simulink model "model — kopia — kopia"  (R2020b)
settings: Solver=VariableStepAuto  StartTime=0.0  StopTime=20000  MaxStep=5  RelTol=1e-3
values from neighbouring files (symbols this model uses):
  A = zeros(2)    [m1 — kopia.m]    (also in model.m)
  B = zeros(2)    [m1 — kopia.m]    (also in model.m)
  Cvg = Cpo*ROo*0.005    (= 14400)    [m1 — kopia.m]    (also in model.m = 14.4)
  Cvw = Cpp*ROp*60    (= 72360)    [m1 — kopia.m]    (also in model.m = 120600)
  dqg = 0 * qg0    (= 0)    [m1 — kopia.m]    (also in model.m = 200)
  dTwew = 0    [m1 — kopia.m]
  dTzew = 3    [m1 — kopia.m]    (also in model.m = 0)
  init_con = [Twew0;Tg0]    [m1 — kopia.m]    (also in model.m = [Twew;Tg])
  k = 5    [m1 — kopia.m]
  Kcg = qg0/(Tg0-Twew0)    (= 100)    [m1 — kopia.m]    (also in model.m)
  Kcw = qg0/(Twew0-Tzew0)    (= 50)    [m1 — kopia.m]    (also in model.m)
  Kp = 0.9*T/(k*T0)    (= 0.46008109478)    [m1 — kopia.m]
  L1 = Kcg    (= 100)    [m1 — kopia.m]    (also in model.m)
  L2 = [Cvg*Kcw,Kcg*Kcw]    [m1 — kopia.m]    (also in model.m)
  L3 = [Cvw,Kcg+Kcw]    [m1 — kopia.m]    (also in model.m)
  L4 = Kcg*Kcw    (= 5000)    [m1 — kopia.m]    (also in model.m)
  M1 = [Cvw*Cvg,Cvg*(Kcg+Kcw)+Cvw*Kcg,Kcw*Kcg]    [m1 — kopia.m]    (also in model.m)
  qg0 = qgN * 1.0    (= 2000)    [m1 — kopia.m]    (also in model.m)
  stepTime = 1000    [m1 — kopia.m]    (also in model.m)
  T = 2521.5    [m1 — kopia.m]
  T0 = 986.5    [m1 — kopia.m]
  Tg = 40    [model.m]
  Ti = 3.33*T0    (= 3285.045)    [m1 — kopia.m]
  Twew = 20    [model.m]
  Twew0 = 20    [m1 — kopia.m]
  Twew_zadana = Twew0    (= 20)    [m1 — kopia.m]
  Tzew0 = TzewN + 0    (= -20)    [m1 — kopia.m]    (also in model.m)
settings Model: OrderedModelArguments=off  Creator=Lab320  LastModifiedBy=Lab320

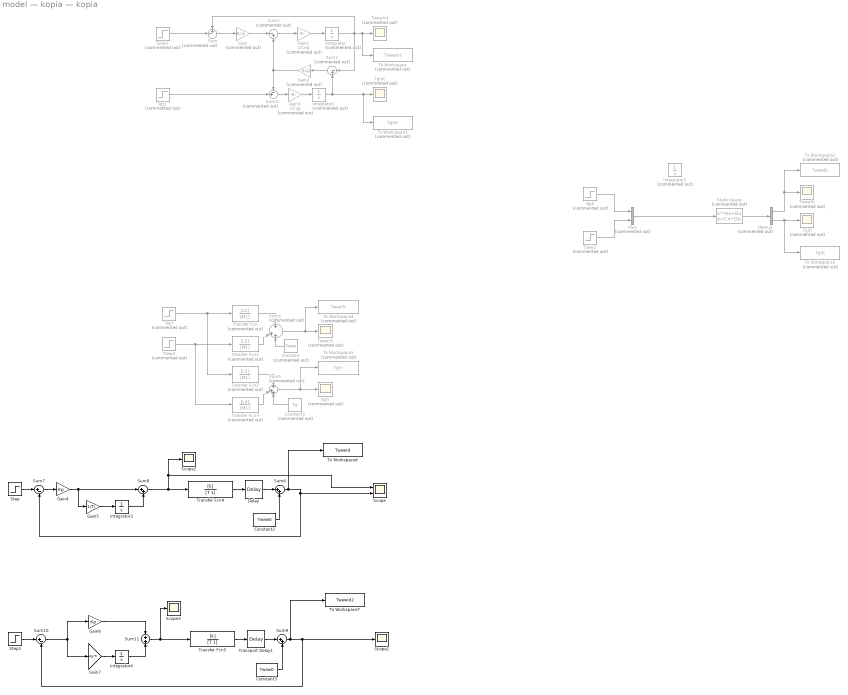
== system model — kopia — kopia ==
  " Delay" : TransportDelay  DelayTime=T0
  Constant : Constant  Commented=on  Value=Twew
  Constant1 : Constant  Commented=on  Value=Tg
  Constant2 : Constant  Value=Twew0
  Constant3 : Constant  Value=Twew0
  Demux : Demux  Commented=on  Outputs=2
  Gain : Gain  Commented=on  Gain=Kcw
  Gain1 : Gain  Commented=on  Gain=1/Cvw
  Gain2 : Gain  Commented=on  Gain=Kcg
  Gain3 : Gain  Commented=on  Gain=1/Cvg
  Gain4 : Gain  Gain=Kp
  Gain5 : Gain  Gain=1/Ti
  Gain6 : Gain  Gain=Kp
  Gain7 : Gain  Gain=Kp/Ti
  Integrator : Integrator  Commented=on  InitialCondition=Twew
  Integrator1 : Integrator  Commented=on  InitialCondition=Tg
  Integrator2 : Integrator  Commented=on
  Integrator3 : Integrator
  Integrator4 : Integrator
  Mux : Mux  Commented=on  Inputs=2
  Qg1 : Step  Commented=on  Time=stepTime  Before=qg0  After=qg0+dqg  SampleTime=0
  Qg2 : Step  Commented=on  Time=stepTime  Before=qg0  After=qg0+dqg  SampleTime=0
  Qg3 : Step  Commented=on  Time=stepTime  After=dqg  SampleTime=0
  Scope : Scope  NumInputPorts=2
  Scope1 : Scope
  Scope2 : Scope
  Scope3 : Scope
  State-Space : StateSpace  Commented=on  A=A  B=B  C=[1,0;0,1]  D=[0,0;0,0]  InitialCondition=init_con
  Step : Step  Time=0  Before=Twew_zadana  After=Twew_zadana+dTwew  SampleTime=0
  Step1 : Step  Time=stepTime  Before=Twew_zadana  After=Twew_zadana+dTwew  SampleTime=0
  Sum : Sum  Commented=on  Inputs=+-|
  Sum1 : Sum  Commented=on  Inputs=|-+
  Sum10 : Sum  Inputs=|+-
  Sum11 : Sum
  Sum2 : Sum  Commented=on  Inputs=|-+
  Sum3 : Sum  Commented=on  Inputs=-+|
  Sum4 : Sum  Commented=on  Inputs=+|++
  Sum5 : Sum  Commented=on  Inputs=+|++
  Sum6 : Sum  Inputs=|++
  Sum7 : Sum  Inputs=|+-
  Sum8 : Sum  Inputs=|++
  Sum9 : Sum  Inputs=|++
  TgInt : Scope  Commented=on
  TgSt : Scope  Commented=on
  TgTr : Scope  Commented=on
  To Workspace : ToWorkspace  Commented=on  VariableName=TwewInt  SaveFormat=Timeseries  SampleTime=-1
  To Workspace1 : ToWorkspace  Commented=on  VariableName=TgInt  SaveFormat=Timeseries  SampleTime=-1
  To Workspace2 : ToWorkspace  Commented=on  VariableName=TwewSt  SaveFormat=Timeseries  SampleTime=-1
  To Workspace3 : ToWorkspace  Commented=on  VariableName=TgSt  SaveFormat=Timeseries  SampleTime=-1
  To Workspace4 : ToWorkspace  Commented=on  VariableName=TwewTr  SaveFormat=Timeseries  SampleTime=-1
  To Workspace5 : ToWorkspace  Commented=on  VariableName=TgTr  SaveFormat=Timeseries  SampleTime=-1
  To Workspace6 : ToWorkspace  VariableName=TwewId  SaveFormat=Timeseries  SampleTime=-1
  To Workspace7 : ToWorkspace  VariableName=TwewId2  SaveFormat=Timeseries  SampleTime=-1
  Transfer Fcn : TransferFcn  Commented=on  Numerator=[L1]  Denominator=[M1]
  Transfer Fcn1 : TransferFcn  Commented=on  Numerator=[L2]  Denominator=[M1]
  Transfer Fcn2 : TransferFcn  Commented=on  Numerator=[L3]  Denominator=[M1]
  Transfer Fcn3 : TransferFcn  Commented=on  Numerator=[L4]  Denominator=[M1]
  Transfer Fcn4 : TransferFcn  Numerator=[k]  Denominator=[T 1]
  Transfer Fcn5 : TransferFcn  Numerator=[k]  Denominator=[T 1]
  Transport Delay1 : TransportDelay  DelayTime=T0
  TwewInt : Scope  Commented=on
  TwewSt : Scope  Commented=on
  TwewTr : Scope  Commented=on
  Tzew1 : Step  Commented=on  Time=stepTime  Before=Tzew0  After=Tzew0+dTzew  SampleTime=0
  Tzew2 : Step  Commented=on  Time=stepTime  Before=Tzew0  After=Tzew0+dTzew  SampleTime=0
  Tzew3 : Step  Commented=on  Time=stepTime  After=dTzew  SampleTime=0
  wires:
  Mux/1 -> State-Space/1
  State-Space/1 -> Demux/1
  Demux/1 -> TwewSt/1, To Workspace2/1
  Demux/2 -> To Workspace3/1, TgSt/1
  Qg2/1 -> Mux/1
  Tzew2/1 -> Mux/2
  Tzew1/1 -> Sum/2
  Sum/1 -> Gain/1
  Gain/1 -> Sum1/1
  Sum1/1 -> Gain1/1
  Gain1/1 -> Integrator/1
  Integrator/1 -> Sum2/1, Sum/1, To Workspace/1, TwewInt/1
  Sum2/1 -> Gain2/1
  Gain2/1 -> Sum3/1, Sum1/2
  Qg1/1 -> Sum3/2
  Sum3/1 -> Gain3/1
  Gain3/1 -> Integrator1/1
  Integrator1/1 -> To Workspace1/1, TgInt/1, Sum2/2
  Qg3/1 -> Transfer Fcn2/1, Transfer Fcn/1
  Tzew3/1 -> Transfer Fcn3/1, Transfer Fcn1/1
  Transfer Fcn/1 -> Sum4/1
  Transfer Fcn1/1 -> Sum4/2
  Transfer Fcn2/1 -> Sum5/1
  Transfer Fcn3/1 -> Sum5/2
  Sum4/1 -> To Workspace4/1, TwewTr/1
  Sum5/1 -> To Workspace5/1, TgTr/1
  Constant/1 -> Sum4/3
  Constant1/1 -> Sum5/3
  Transfer Fcn4/1 -> " Delay"/1
  " Delay"/1 -> Sum6/1
  Constant2/1 -> Sum6/2
  Sum6/1 -> To Workspace6/1, Sum7/2, Scope/2
  Step/1 -> Sum7/1
  Sum7/1 -> Gain4/1
  Gain4/1 -> Sum8/1, Gain5/1
  Gain5/1 -> Integrator3/1
  Integrator3/1 -> Sum8/2
  Sum8/1 -> Scope/1, Scope2/1, Transfer Fcn4/1
  Sum11/1 -> Scope3/1, Transfer Fcn5/1
  Sum10/1 -> Gain7/1, Gain6/1
  Step1/1 -> Sum10/1
  Sum9/1 -> Scope1/1, Sum10/2, To Workspace7/1
  Constant3/1 -> Sum9/2
  Transport Delay1/1 -> Sum9/1
  Transfer Fcn5/1 -> Transport Delay1/1
  Gain7/1 -> Integrator4/1
  Integrator4/1 -> Sum11/2
  Gain6/1 -> Sum11/1
